simulink library "myLibrary"  (R2023b)
settings: Solver=VariableStepAuto  StartTime=0.0  StopTime=10.0  RelTol=1e-3
undefined symbols (not defined in the file): Cac_n1, ctrl1, Da, Discrete, dtha, ee_sli_rtmsupport, FA, gcbh, Ha, Ini, init_DCline, init_IPC, init_line, init_load, init_SG, init_shunt, init_TH, init_trafo, init_VSC, initMachineBlocks, Ka, Lf, Llkd_pu, Llkq1_pu, magnitude, NET, P, plots_step, q0, Rac_n1, Radd, Rkd_pu, Rkq1_pu, Rload_add, sim_config, sps_rtmsupport, spsSteamTurbineModel, T_DC_NET, T_global, T_IPC, T_load, T_NET, T_SG, T_shunt, T_STATCOM, T_TH, T_trafo, T_VSC, Ts, tstep, Udiff_a, V1
libraries: spsSeriesRLCBranchLib x105, eeGeneralControl x72, $bdroot x70, spsCurrentMeasurementLib x48, spsParallelRLCBranchLib x39, spsVoltageMeasurementLib x33, spsControlledVoltageSourceLib x27, spsFirstOrderFilterLib x16, dspsigops x6, spsThreePhaseVIMeasurementLib x5, spsPLL3phLib x4, spsThreePhaseBreakerLib x3
(part 2 of 12)

== system myLibrary/HVDC_line ==
  Current Measurement : spsCurrentMeasurementLib/Current Measurement  PhasorSimulation=off  OutputType=Complex  PSBequivalent=0
  Current Measurement1 : Subsystem  DialogController=POWERSYS.PowerSysDialog  LoadFcn=sps_rtmsupport('LoadFcn',gcbh);  StartFcn=sps_rtmsupport('StartFcn',gcbh);  StopFcn=sps_rtmsupport('StopFcn',gcbh);  mask(Current Measurement){PhasorSimulation=off, OutputType=Complex, PSBequivalent=0}
      mask prompts: PhasorSimulation "Phasor simulation"; OutputType "Output signal :"; PSBequivalent "Equivalent circuit"
      mask help: Ideal current measurement. The Output signal parameter is disabled when the block is not used in a phasor simulation. The phasor simulation is activated by a Powergui block placed in the model.
      mask init:
      | block = gcb;
      | powericon('psbloadfunction',block,'Measurement Block','Initialize');
      | WantBlockChoice = powericon('MeasurementBlockInit',block);
      | powericon('SetInternalModels','set',block,WantBlockChoice);
      | power_initmask();
      settings: LibrarySourceBlock=sps_lib/Sensors and Measurements/Current Measurement  CopyFcn=sps_rtmsupport('CopyFcn',gcbh); powericon('psbloadfunction',gcb,'Measurement Block','UpdateGotoTag');  DeleteFcn=sps_rtmsupport('DeleteFcn',gcbh);  UndoDeleteFcn=sps_rtmsupport('UndoDeleteFcn',gcbh);  ModelCloseFcn=sps_rtmsupport('ModelCloseFcn',gcbh);  PreSaveFcn=sps_rtmsupport('PreSaveFcn',gcbh);  PostSaveFcn=sps_rtmsupport('PostSaveFcn',gcbh);  PreCopyFcn=sps_rtmsupport('PreCopyFcn',gcbh);  OpenFcn=sps_rtmsupport('OpenFcn',gcbh, [1 -2]);  CloseFcn=sps_rtmsupport('CloseFcn',gcbh);  PreDeleteFcn=sps_rtmsupport('PreDeleteFcn',gcbh);
      settings: NameChangeFcn=|
      | sps_rtmsupport('NameChangeFcn',gcbh);
      | powericon('SetNewGotoTag',[gcb,'/source'],-2);
      mask Help: helpview(psbhelp);
      mask TypeOptions OutputType: Complex | Real-Imag | Magnitude-Angle | Magnitude
  Current Measurement2 : Subsystem  DialogController=POWERSYS.PowerSysDialog  LoadFcn=sps_rtmsupport('LoadFcn',gcbh);  StartFcn=sps_rtmsupport('StartFcn',gcbh);  StopFcn=sps_rtmsupport('StopFcn',gcbh);  mask(Current Measurement){PhasorSimulation=off, OutputType=Complex, PSBequivalent=0}
      mask prompts: PhasorSimulation "Phasor simulation"; OutputType "Output signal :"; PSBequivalent "Equivalent circuit"
      mask help: Ideal current measurement. The Output signal parameter is disabled when the block is not used in a phasor simulation. The phasor simulation is activated by a Powergui block placed in the model.
      mask init: same as myLibrary/HVDC_line/Current Measurement1
      settings: LibrarySourceBlock=sps_lib/Sensors and Measurements/Current Measurement  CopyFcn=sps_rtmsupport('CopyFcn',gcbh); powericon('psbloadfunction',gcb,'Measurement Block','UpdateGotoTag');  DeleteFcn=sps_rtmsupport('DeleteFcn',gcbh);  UndoDeleteFcn=sps_rtmsupport('UndoDeleteFcn',gcbh);  ModelCloseFcn=sps_rtmsupport('ModelCloseFcn',gcbh);  PreSaveFcn=sps_rtmsupport('PreSaveFcn',gcbh);  PostSaveFcn=sps_rtmsupport('PostSaveFcn',gcbh);  PreCopyFcn=sps_rtmsupport('PreCopyFcn',gcbh);  OpenFcn=sps_rtmsupport('OpenFcn',gcbh, [1 -2]);  CloseFcn=sps_rtmsupport('CloseFcn',gcbh);  PreDeleteFcn=sps_rtmsupport('PreDeleteFcn',gcbh);
      settings: NameChangeFcn=|
      | sps_rtmsupport('NameChangeFcn',gcbh);
      | powericon('SetNewGotoTag',[gcb,'/source'],-2);
      mask Help: helpview(psbhelp);
      mask TypeOptions OutputType: Complex | Real-Imag | Magnitude-Angle | Magnitude
  Scope : Scope  NumInputPorts=3
  Series RLC Branch1 : PMComponent  DialogController=POWERSYS.PowerSysDialog  LoadFcn=sps_rtmsupport('LoadFcn',gcbh);  StartFcn=sps_rtmsupport('StartFcn',gcbh);  StopFcn=sps_rtmsupport('StopFcn',gcbh);  PhysicalDomain=powersysdomain  LeftPortType=p1  RightPortType=p1  LConnTagsString=__new0  RConnTagsString=__new0  mask(Series RLC Branch){BranchType=C, Resistance=1, Inductance=1e-3, SetiL0=off, InitialCurrent=0, Capacitance=T.C, Setx0=on, InitialVoltage=ini.V1, Measurements=None}
      mask prompts: BranchType "Branch type:"; Resistance "Resistance (Ohms):"; Inductance "Inductance (H):"; SetiL0 "Set the initial inductor current"; InitialCurrent "Inductor initial current (A):"; Capacitance "Capacitance (F):"; Setx0 "Set the initial capacitor voltage"; InitialVoltage "Capacitor initial voltage (V):"
      mask help:
      | Implements a series branch of RLC elements.
      | Use the 'Branch type' parameter to add or remove elements from the branch.
      mask init:
      | [s1,s2,s3,s4,r1,r2,l1,l2,c1,c2,c3,c4] = powericon('Series RLC Branch',Resistance,Inductance,Capacitance,BranchType);
      | powericon('RLCCback',gcb)
      | power_initmask();
      settings: LibrarySourceBlock=spsSeriesRLCBranchLib/Series RLC Branch  CopyFcn=sps_rtmsupport('CopyFcn',gcbh);  DeleteFcn=sps_rtmsupport('DeleteFcn',gcbh);  UndoDeleteFcn=sps_rtmsupport('UndoDeleteFcn',gcbh);  ModelCloseFcn=sps_rtmsupport('ModelCloseFcn',gcbh);  PreSaveFcn=sps_rtmsupport('PreSaveFcn',gcbh);  PostSaveFcn=sps_rtmsupport('PostSaveFcn',gcbh);  NameChangeFcn=sps_rtmsupport('NameChangeFcn',gcbh);  PreCopyFcn=sps_rtmsupport('PreCopyFcn',gcbh);  OpenFcn=sps_rtmsupport('OpenFcn',gcbh, [1 4 7 9]);  CloseFcn=sps_rtmsupport('CloseFcn',gcbh);  PreDeleteFcn=sps_rtmsupport('PreDeleteFcn',gcbh);
      mask Help: helpview(psbhelp);
      mask TypeOptions BranchType: RLC | R | L | C | RL | RC | LC | Open circuit
      mask Callback BranchType: powericon('RLCCback',gcb)
      mask Callback Resistance: powericon('RLCCback',gcb)
      mask Callback Inductance: powericon('RLCCback',gcb)
      mask Callback SetiL0: powericon('RLCCback',gcb)
      mask Callback Capacitance: powericon('RLCCback',gcb)
      mask Callback Setx0: powericon('RLCCback',gcb)
      mask TypeOptions Measurements: None | Branch voltage | Branch current | Branch voltage and current
      mask Display:
      | plot(s1,s2,s3,s4,r1,r2*1.5,l1,l2*1.5,c1,c2*1.5,c3,c4*1.5)
      | color('red')
      | port_label('LConn',1,'+')
  Series RLC Branch4 : spsSeriesRLCBranchLib/Series RLC Branch  LConnTagsString=__new0  RConnTagsString=__new0  BranchType=C  Resistance=1  Inductance=1e-3  SetiL0=off  InitialCurrent=0  Capacitance=T.C  Setx0=on  InitialVoltage=ini.V2  Measurements=None
  Series RLC Branch6 : spsSeriesRLCBranchLib/Series RLC Branch  LConnTagsString=__new0  RConnTagsString=__new0  BranchType=RL  Resistance=T.Ra  Inductance=T.La  SetiL0=on  InitialCurrent=ini.Ia  Capacitance=P.C  Setx0=on  InitialVoltage=P.C  Measurements=None
  Series RLC Branch7 : spsSeriesRLCBranchLib/Series RLC Branch  LConnTagsString=__new0  RConnTagsString=__new0  BranchType=RL  Resistance=T.Rc  Inductance=T.Lc  SetiL0=on  InitialCurrent=ini.Ic  Capacitance=P.C  Setx0=on  InitialVoltage=P.C  Measurements=None
  Series RLC Branch8 : spsSeriesRLCBranchLib/Series RLC Branch  LConnTagsString=__new0  RConnTagsString=__new0  BranchType=RL  Resistance=T.Rb  Inductance=T.Lb  SetiL0=on  InitialCurrent=ini.Ib  Capacitance=P.C  Setx0=on  InitialVoltage=P.C  Measurements=None
  Vdc+2 : PMIOPort  Side=Right
  Vcd+1 : PMIOPort  Port=2  Side=Left
  Vdc-1 : PMIOPort  Port=3  Side=Left
  Vdc-2 : PMIOPort  Port=4  Side=Right
  wires:
  Current Measurement/1 -> Scope/1
  Current Measurement1/1(i) -> Scope/2
  Current Measurement2/1(i) -> Scope/3
  connections:
  Series RLC Branch4/LConn1 -- Current Measurement1/RConn1 -- Current Measurement/RConn1 -- Current Measurement2/RConn1 -- Vdc+2/RConn1
  Series RLC Branch1/LConn1 -- Vcd+1/RConn1 -- Series RLC Branch7/LConn1 -- Series RLC Branch6/LConn1 -- Series RLC Branch8/LConn1
  Vdc-1/RConn1 -- Vdc-2/RConn1 -- Series RLC Branch4/RConn1 -- Series RLC Branch1/RConn1
  Current Measurement/LConn1 -- Series RLC Branch6/RConn1
  Series RLC Branch8/RConn1 -- Current Measurement1/LConn1
  Current Measurement2/LConn1 -- Series RLC Branch7/RConn1

== system myLibrary/Load ==
  Parallel RLC Branch : spsParallelRLCBranchLib/Parallel RLC Branch  LConnTagsString=a  RConnTagsString=__new0  BranchType=R  Resistance=T.R  Inductance=P.L  SetiL0=on  InitialCurrent=Ini.Ia*10  Capacitance=1e-6  Setx0=off  InitialVoltage=0  Measurements=None
  Parallel RLC Branch1 : spsParallelRLCBranchLib/Parallel RLC Branch  LConnTagsString=a  RConnTagsString=__new0  BranchType=R  Resistance=T.R  Inductance=P.L  SetiL0=on  InitialCurrent=Ini.Ia*10  Capacitance=1e-6  Setx0=off  InitialVoltage=0  Measurements=None
  Parallel RLC Branch2 : spsParallelRLCBranchLib/Parallel RLC Branch  LConnTagsString=a  RConnTagsString=__new0  BranchType=L  Resistance=P.R  Inductance=T.L  SetiL0=on  InitialCurrent=ini.Ib  Capacitance=1e-6  Setx0=off  InitialVoltage=0  Measurements=None
  Parallel RLC Branch3 : spsParallelRLCBranchLib/Parallel RLC Branch  LConnTagsString=a  RConnTagsString=__new0  BranchType=L  Resistance=P.R  Inductance=T.L  SetiL0=on  InitialCurrent=ini.Ia  Capacitance=1e-6  Setx0=off  InitialVoltage=0  Measurements=None
  Parallel RLC Branch4 : spsParallelRLCBranchLib/Parallel RLC Branch  LConnTagsString=a  RConnTagsString=__new0  BranchType=R  Resistance=T.R  Inductance=P.L  SetiL0=on  InitialCurrent=Ini.Ia*10  Capacitance=1e-6  Setx0=off  InitialVoltage=0  Measurements=None
  Parallel RLC Branch5 : spsParallelRLCBranchLib/Parallel RLC Branch  LConnTagsString=a  RConnTagsString=__new0  BranchType=L  Resistance=P.R  Inductance=T.L  SetiL0=on  InitialCurrent=ini.Ic  Capacitance=1e-6  Setx0=off  InitialVoltage=0  Measurements=None
  A : PMIOPort  Side=Left
  B : PMIOPort  Port=2  Side=Left
  C : PMIOPort  Port=3  Side=Left
  connections:
  Parallel RLC Branch2/LConn1 -- Parallel RLC Branch1/RConn1 -- Parallel RLC Branch3/LConn1 -- Parallel RLC Branch/RConn1 -- Parallel RLC Branch4/RConn1 -- Parallel RLC Branch5/LConn1
  A/RConn1 -- Parallel RLC Branch3/RConn1 -- Parallel RLC Branch/LConn1
  Parallel RLC Branch1/LConn1 -- B/RConn1 -- Parallel RLC Branch2/RConn1
  C/RConn1 -- Parallel RLC Branch5/RConn1 -- Parallel RLC Branch4/LConn1

== system myLibrary/LoadC ==
  Parallel RLC Branch : spsParallelRLCBranchLib/Parallel RLC Branch  LConnTagsString=a  RConnTagsString=__new0  BranchType=R  Resistance=T.R  Inductance=P.L  SetiL0=on  InitialCurrent=Ini.Ia*10  Capacitance=1e-6  Setx0=off  InitialVoltage=0  Measurements=None
  Parallel RLC Branch1 : spsParallelRLCBranchLib/Parallel RLC Branch  LConnTagsString=a  RConnTagsString=__new0  BranchType=R  Resistance=T.R  Inductance=P.L  SetiL0=on  InitialCurrent=Ini.Ia*10  Capacitance=1e-6  Setx0=off  InitialVoltage=0  Measurements=None
  Parallel RLC Branch2 : spsParallelRLCBranchLib/Parallel RLC Branch  LConnTagsString=a  RConnTagsString=__new0  BranchType=C  Resistance=T.R  Inductance=P.L  SetiL0=on  InitialCurrent=Ini.Ia*10  Capacitance=T.C  Setx0=on  InitialVoltage=ini.Va  Measurements=None
  Parallel RLC Branch3 : spsParallelRLCBranchLib/Parallel RLC Branch  LConnTagsString=a  RConnTagsString=__new0  BranchType=C  Resistance=T.R  Inductance=P.L  SetiL0=on  InitialCurrent=Ini.Ia*10  Capacitance=T.C  Setx0=on  InitialVoltage=ini.Vb  Measurements=None
  Parallel RLC Branch4 : spsParallelRLCBranchLib/Parallel RLC Branch  LConnTagsString=a  RConnTagsString=__new0  BranchType=R  Resistance=T.R  Inductance=P.L  SetiL0=on  InitialCurrent=Ini.Ia*10  Capacitance=1e-6  Setx0=off  InitialVoltage=0  Measurements=None
  Parallel RLC Branch5 : spsParallelRLCBranchLib/Parallel RLC Branch  LConnTagsString=a  RConnTagsString=__new0  BranchType=C  Resistance=T.R  Inductance=P.L  SetiL0=on  InitialCurrent=Ini.Ia*10  Capacitance=T.C  Setx0=on  InitialVoltage=ini.Vc  Measurements=None
  A : PMIOPort  Side=Left
  B : PMIOPort  Port=2  Side=Left
  C : PMIOPort  Port=3  Side=Left
  connections:
  Parallel RLC Branch1/RConn1 -- Parallel RLC Branch3/RConn1 -- Parallel RLC Branch2/RConn1 -- Parallel RLC Branch/RConn1 -- Parallel RLC Branch5/RConn1 -- Parallel RLC Branch4/RConn1
  A/RConn1 -- Parallel RLC Branch2/LConn1 -- Parallel RLC Branch/LConn1
  Parallel RLC Branch1/LConn1 -- Parallel RLC Branch3/LConn1 -- B/RConn1
  C/RConn1 -- Parallel RLC Branch5/LConn1 -- Parallel RLC Branch4/LConn1

== system myLibrary/LoadC_Rstep ==
  Parallel RLC Branch : spsParallelRLCBranchLib/Parallel RLC Branch  LConnTagsString=a  RConnTagsString=__new0  BranchType=R  Resistance=T.R  Inductance=P.L  SetiL0=on  InitialCurrent=Ini.Ia*10  Capacitance=1e-6  Setx0=off  InitialVoltage=0  Measurements=None
  Parallel RLC Branch1 : spsParallelRLCBranchLib/Parallel RLC Branch  LConnTagsString=a  RConnTagsString=__new0  BranchType=R  Resistance=T.R  Inductance=P.L  SetiL0=on  InitialCurrent=Ini.Ia*10  Capacitance=1e-6  Setx0=off  InitialVoltage=0  Measurements=None
  Parallel RLC Branch10 : spsParallelRLCBranchLib/Parallel RLC Branch  LConnTagsString=a  RConnTagsString=__new0  BranchType=R  Resistance=Rload_add  Inductance=P.L  SetiL0=on  InitialCurrent=Ini.Ia*10  Capacitance=1e-6  Setx0=off  InitialVoltage=0  Measurements=None
  Parallel RLC Branch2 : spsParallelRLCBranchLib/Parallel RLC Branch  LConnTagsString=a  RConnTagsString=__new0  BranchType=C  Resistance=T.R  Inductance=P.L  SetiL0=on  InitialCurrent=Ini.Ia*10  Capacitance=T.C  Setx0=on  InitialVoltage=ini.Va  Measurements=None
  Parallel RLC Branch3 : spsParallelRLCBranchLib/Parallel RLC Branch  LConnTagsString=a  RConnTagsString=__new0  BranchType=C  Resistance=T.R  Inductance=P.L  SetiL0=on  InitialCurrent=Ini.Ia*10  Capacitance=T.C  Setx0=on  InitialVoltage=ini.Vb  Measurements=None
  Parallel RLC Branch4 : spsParallelRLCBranchLib/Parallel RLC Branch  LConnTagsString=a  RConnTagsString=__new0  BranchType=R  Resistance=T.R  Inductance=P.L  SetiL0=on  InitialCurrent=Ini.Ia*10  Capacitance=1e-6  Setx0=off  InitialVoltage=0  Measurements=None
  Parallel RLC Branch5 : spsParallelRLCBranchLib/Parallel RLC Branch  LConnTagsString=a  RConnTagsString=__new0  BranchType=C  Resistance=T.R  Inductance=P.L  SetiL0=on  InitialCurrent=Ini.Ia*10  Capacitance=T.C  Setx0=on  InitialVoltage=ini.Vc  Measurements=None
  Parallel RLC Branch6 : spsParallelRLCBranchLib/Parallel RLC Branch  LConnTagsString=a  RConnTagsString=__new0  BranchType=R  Resistance=Rload_add  Inductance=P.L  SetiL0=on  InitialCurrent=Ini.Ia*10  Capacitance=1e-6  Setx0=off  InitialVoltage=0  Measurements=None
  Parallel RLC Branch7 : spsParallelRLCBranchLib/Parallel RLC Branch  LConnTagsString=a  RConnTagsString=__new0  BranchType=R  Resistance=Rload_add  Inductance=P.L  SetiL0=on  InitialCurrent=Ini.Ia*10  Capacitance=1e-6  Setx0=off  InitialVoltage=0  Measurements=None
  Three-Phase Breaker : spsThreePhaseBreakerLib/Three-Phase Breaker  InitialState=open  SwitchA=on  SwitchB=on  SwitchC=on  SwitchTimes=[tstep 1e6]  External=off  BreakerResistance=1e-10  SnubberResistance=inf  SnubberCapacitance=inf  Measurements=None
  A : PMIOPort  Side=Left
  B : PMIOPort  Port=2  Side=Left
  C : PMIOPort  Port=3  Side=Left
  connections:
  Three-Phase Breaker/RConn3 -- Parallel RLC Branch10/LConn1
  Three-Phase Breaker/RConn2 -- Parallel RLC Branch7/LConn1
  Three-Phase Breaker/RConn1 -- Parallel RLC Branch6/LConn1
  Parallel RLC Branch10/RConn1 -- Parallel RLC Branch7/RConn1 -- Parallel RLC Branch6/RConn1 -- Parallel RLC Branch4/RConn1 -- Parallel RLC Branch2/RConn1 -- Parallel RLC Branch/RConn1 -- Parallel RLC Branch3/RConn1 -- Parallel RLC Branch1/RConn1 -- Parallel RLC Branch5/RConn1
  Parallel RLC Branch4/LConn1 -- Parallel RLC Branch5/LConn1 -- C/RConn1 -- Three-Phase Breaker/LConn3
  Parallel RLC Branch1/LConn1 -- Parallel RLC Branch3/LConn1 -- B/RConn1 -- Three-Phase Breaker/LConn2
  Parallel RLC Branch/LConn1 -- Parallel RLC Branch2/LConn1 -- A/RConn1 -- Three-Phase Breaker/LConn1

== system myLibrary/Load_R ==
  Parallel RLC Branch : spsParallelRLCBranchLib/Parallel RLC Branch  LConnTagsString=a  RConnTagsString=__new0  BranchType=R  Resistance=T.R  Inductance=P.L  SetiL0=on  InitialCurrent=Ini.Ia*10  Capacitance=1e-6  Setx0=off  InitialVoltage=0  Measurements=None
  Parallel RLC Branch1 : spsParallelRLCBranchLib/Parallel RLC Branch  LConnTagsString=a  RConnTagsString=__new0  BranchType=R  Resistance=T.R  Inductance=P.L  SetiL0=on  InitialCurrent=Ini.Ia*10  Capacitance=1e-6  Setx0=off  InitialVoltage=0  Measurements=None
  Parallel RLC Branch4 : spsParallelRLCBranchLib/Parallel RLC Branch  LConnTagsString=a  RConnTagsString=__new0  BranchType=R  Resistance=T.R  Inductance=P.L  SetiL0=on  InitialCurrent=Ini.Ia*10  Capacitance=1e-6  Setx0=off  InitialVoltage=0  Measurements=None
  A : PMIOPort  Side=Left
  B : PMIOPort  Port=2  Side=Left
  C : PMIOPort  Port=3  Side=Left
  connections:
  Parallel RLC Branch1/RConn1 -- Parallel RLC Branch4/RConn1 -- Parallel RLC Branch/RConn1
  Parallel RLC Branch/LConn1 -- A/RConn1
  Parallel RLC Branch1/LConn1 -- B/RConn1
  Parallel RLC Branch4/LConn1 -- C/RConn1

== system myLibrary/Load_R_Rstep ==
  Parallel RLC Branch : spsParallelRLCBranchLib/Parallel RLC Branch  LConnTagsString=a  RConnTagsString=__new0  BranchType=R  Resistance=T.R  Inductance=P.L  SetiL0=on  InitialCurrent=Ini.Ia*10  Capacitance=1e-6  Setx0=off  InitialVoltage=0  Measurements=None
  Parallel RLC Branch1 : spsParallelRLCBranchLib/Parallel RLC Branch  LConnTagsString=a  RConnTagsString=__new0  BranchType=R  Resistance=T.R  Inductance=P.L  SetiL0=on  InitialCurrent=Ini.Ia*10  Capacitance=1e-6  Setx0=off  InitialVoltage=0  Measurements=None
  Parallel RLC Branch10 : spsParallelRLCBranchLib/Parallel RLC Branch  LConnTagsString=a  RConnTagsString=__new0  BranchType=R  Resistance=Rload_add  Inductance=P.L  SetiL0=on  InitialCurrent=Ini.Ia*10  Capacitance=1e-6  Setx0=off  InitialVoltage=0  Measurements=None
  Parallel RLC Branch4 : spsParallelRLCBranchLib/Parallel RLC Branch  LConnTagsString=a  RConnTagsString=__new0  BranchType=R  Resistance=T.R  Inductance=P.L  SetiL0=on  InitialCurrent=Ini.Ia*10  Capacitance=1e-6  Setx0=off  InitialVoltage=0  Measurements=None
  Parallel RLC Branch6 : spsParallelRLCBranchLib/Parallel RLC Branch  LConnTagsString=a  RConnTagsString=__new0  BranchType=R  Resistance=Rload_add  Inductance=P.L  SetiL0=on  InitialCurrent=Ini.Ia*10  Capacitance=1e-6  Setx0=off  InitialVoltage=0  Measurements=None
  Parallel RLC Branch7 : spsParallelRLCBranchLib/Parallel RLC Branch  LConnTagsString=a  RConnTagsString=__new0  BranchType=R  Resistance=Rload_add  Inductance=P.L  SetiL0=on  InitialCurrent=Ini.Ia*10  Capacitance=1e-6  Setx0=off  InitialVoltage=0  Measurements=None
  Three-Phase Breaker : spsThreePhaseBreakerLib/Three-Phase Breaker  InitialState=open  SwitchA=on  SwitchB=on  SwitchC=on  SwitchTimes=[tstep 1e6]  External=off  BreakerResistance=1e-10  SnubberResistance=inf  SnubberCapacitance=inf  Measurements=None
  A : PMIOPort  Side=Left
  B : PMIOPort  Port=2  Side=Left
  C : PMIOPort  Port=3  Side=Left
  connections:
  Three-Phase Breaker/LConn1 -- Parallel RLC Branch/LConn1 -- A/RConn1
  Parallel RLC Branch1/LConn1 -- Three-Phase Breaker/LConn2 -- B/RConn1
  Three-Phase Breaker/LConn3 -- Parallel RLC Branch4/LConn1 -- C/RConn1
  Parallel RLC Branch1/RConn1 -- Parallel RLC Branch/RConn1 -- Parallel RLC Branch6/RConn1 -- Parallel RLC Branch7/RConn1 -- Parallel RLC Branch10/RConn1 -- Parallel RLC Branch4/RConn1
  Three-Phase Breaker/RConn1 -- Parallel RLC Branch6/LConn1
  Three-Phase Breaker/RConn2 -- Parallel RLC Branch7/LConn1
  Three-Phase Breaker/RConn3 -- Parallel RLC Branch10/LConn1

== system myLibrary/Load_Rstep ==
  Parallel RLC Branch : spsParallelRLCBranchLib/Parallel RLC Branch  LConnTagsString=a  RConnTagsString=__new0  BranchType=R  Resistance=T.R  Inductance=P.L  SetiL0=on  InitialCurrent=Ini.Ia*10  Capacitance=1e-6  Setx0=off  InitialVoltage=0  Measurements=None
  Parallel RLC Branch1 : spsParallelRLCBranchLib/Parallel RLC Branch  LConnTagsString=a  RConnTagsString=__new0  BranchType=R  Resistance=T.R  Inductance=P.L  SetiL0=on  InitialCurrent=Ini.Ia*10  Capacitance=1e-6  Setx0=off  InitialVoltage=0  Measurements=None
  Parallel RLC Branch10 : spsParallelRLCBranchLib/Parallel RLC Branch  LConnTagsString=a  RConnTagsString=__new0  BranchType=R  Resistance=Rload_add  Inductance=P.L  SetiL0=on  InitialCurrent=Ini.Ia*10  Capacitance=1e-6  Setx0=off  InitialVoltage=0  Measurements=None
  Parallel RLC Branch2 : spsParallelRLCBranchLib/Parallel RLC Branch  LConnTagsString=a  RConnTagsString=__new0  BranchType=L  Resistance=P.R  Inductance=T.L  SetiL0=on  InitialCurrent=ini.Ib  Capacitance=1e-6  Setx0=off  InitialVoltage=0  Measurements=None
  Parallel RLC Branch3 : spsParallelRLCBranchLib/Parallel RLC Branch  LConnTagsString=a  RConnTagsString=__new0  BranchType=L  Resistance=P.R  Inductance=T.L  SetiL0=on  InitialCurrent=ini.Ia  Capacitance=1e-6  Setx0=off  InitialVoltage=0  Measurements=None
  Parallel RLC Branch4 : spsParallelRLCBranchLib/Parallel RLC Branch  LConnTagsString=a  RConnTagsString=__new0  BranchType=R  Resistance=T.R  Inductance=P.L  SetiL0=on  InitialCurrent=Ini.Ia*10  Capacitance=1e-6  Setx0=off  InitialVoltage=0  Measurements=None
  Parallel RLC Branch5 : spsParallelRLCBranchLib/Parallel RLC Branch  LConnTagsString=a  RConnTagsString=__new0  BranchType=L  Resistance=P.R  Inductance=T.L  SetiL0=on  InitialCurrent=ini.Ic  Capacitance=1e-6  Setx0=off  InitialVoltage=0  Measurements=None
  Parallel RLC Branch6 : spsParallelRLCBranchLib/Parallel RLC Branch  LConnTagsString=a  RConnTagsString=__new0  BranchType=R  Resistance=Rload_add  Inductance=P.L  SetiL0=on  InitialCurrent=Ini.Ia*10  Capacitance=1e-6  Setx0=off  InitialVoltage=0  Measurements=None
  Parallel RLC Branch7 : spsParallelRLCBranchLib/Parallel RLC Branch  LConnTagsString=a  RConnTagsString=__new0  BranchType=R  Resistance=Rload_add  Inductance=P.L  SetiL0=on  InitialCurrent=Ini.Ia*10  Capacitance=1e-6  Setx0=off  InitialVoltage=0  Measurements=None
  Three-Phase Breaker : spsThreePhaseBreakerLib/Three-Phase Breaker  InitialState=open  SwitchA=on  SwitchB=on  SwitchC=on  SwitchTimes=[tstep 1e6]  External=off  BreakerResistance=1e-10  SnubberResistance=inf  SnubberCapacitance=inf  Measurements=None
  A : PMIOPort  Side=Left
  B : PMIOPort  Port=2  Side=Left
  C : PMIOPort  Port=3  Side=Left
  connections:
  Three-Phase Breaker/LConn1 -- A/RConn1 -- Parallel RLC Branch3/RConn1 -- Parallel RLC Branch/LConn1
  Parallel RLC Branch1/LConn1 -- Three-Phase Breaker/LConn2 -- B/RConn1 -- Parallel RLC Branch2/RConn1
  Three-Phase Breaker/LConn3 -- C/RConn1 -- Parallel RLC Branch5/RConn1 -- Parallel RLC Branch4/LConn1
  Parallel RLC Branch2/LConn1 -- Parallel RLC Branch1/RConn1 -- Parallel RLC Branch3/LConn1 -- Parallel RLC Branch/RConn1 -- Parallel RLC Branch4/RConn1 -- Parallel RLC Branch5/LConn1 -- Parallel RLC Branch6/RConn1 -- Parallel RLC Branch7/RConn1 -- Parallel RLC Branch10/RConn1
  Three-Phase Breaker/RConn1 -- Parallel RLC Branch6/LConn1
  Three-Phase Breaker/RConn2 -- Parallel RLC Branch7/LConn1
  Three-Phase Breaker/RConn3 -- Parallel RLC Branch10/LConn1

== system myLibrary/PI_line ==
  Series RLC Branch : spsSeriesRLCBranchLib/Series RLC Branch  LConnTagsString=__new0  RConnTagsString=__new0  BranchType=C  Resistance=1  Inductance=1e-3  SetiL0=off  InitialCurrent=0  Capacitance=T.C  Setx0=on  InitialVoltage=ini.Va1  Measurements=None
  Series RLC Branch1 : spsSeriesRLCBranchLib/Series RLC Branch  LConnTagsString=__new0  RConnTagsString=__new0  BranchType=C  Resistance=1  Inductance=1e-3  SetiL0=off  InitialCurrent=0  Capacitance=T.C  Setx0=on  InitialVoltage=ini.Vb1  Measurements=None
  Series RLC Branch2 : spsSeriesRLCBranchLib/Series RLC Branch  LConnTagsString=__new0  RConnTagsString=__new0  BranchType=C  Resistance=1  Inductance=1e-3  SetiL0=off  InitialCurrent=0  Capacitance=T.C  Setx0=on  InitialVoltage=ini.Vc1  Measurements=None
  Series RLC Branch3 : spsSeriesRLCBranchLib/Series RLC Branch  LConnTagsString=__new0  RConnTagsString=__new0  BranchType=C  Resistance=1  Inductance=1e-3  SetiL0=off  InitialCurrent=0  Capacitance=T.C  Setx0=on  InitialVoltage=ini.Va2  Measurements=None
  Series RLC Branch4 : spsSeriesRLCBranchLib/Series RLC Branch  LConnTagsString=__new0  RConnTagsString=__new0  BranchType=C  Resistance=1  Inductance=1e-3  SetiL0=off  InitialCurrent=0  Capacitance=T.C  Setx0=on  InitialVoltage=ini.Vb2  Measurements=None
  Series RLC Branch5 : spsSeriesRLCBranchLib/Series RLC Branch  LConnTagsString=__new0  RConnTagsString=__new0  BranchType=C  Resistance=1  Inductance=1e-3  SetiL0=off  InitialCurrent=0  Capacitance=T.C  Setx0=on  InitialVoltage=ini.Vc2  Measurements=None
  Series RLC Branch6 : spsSeriesRLCBranchLib/Series RLC Branch  LConnTagsString=__new0  RConnTagsString=__new0  BranchType=RL  Resistance=T.R  Inductance=T.L  SetiL0=off  InitialCurrent=ini.Ia  Capacitance=P.C  Setx0=on  InitialVoltage=P.C  Measurements=None
  Series RLC Branch7 : spsSeriesRLCBranchLib/Series RLC Branch  LConnTagsString=__new0  RConnTagsString=__new0  BranchType=RL  Resistance=T.R  Inductance=T.L  SetiL0=on  InitialCurrent=ini.Ic  Capacitance=P.C  Setx0=on  InitialVoltage=P.C  Measurements=None
  Series RLC Branch8 : spsSeriesRLCBranchLib/Series RLC Branch  LConnTagsString=__new0  RConnTagsString=__new0  BranchType=RL  Resistance=T.R  Inductance=T.L  SetiL0=on  InitialCurrent=ini.Ib  Capacitance=P.C  Setx0=on  InitialVoltage=P.C  Measurements=None
  A1 : PMIOPort  Side=Left
  B1 : PMIOPort  Port=2  Side=Left
  C1 : PMIOPort  Port=3  Side=Left
  A2 : PMIOPort  Port=4  Side=Right
  B2 : PMIOPort  Port=5  Side=Right
  C2 : PMIOPort  Port=6  Side=Right
  connections:
  C2/RConn1 -- Series RLC Branch7/RConn1 -- Series RLC Branch5/LConn1
  B2/RConn1 -- Series RLC Branch8/RConn1 -- Series RLC Branch4/LConn1
  Series RLC Branch3/LConn1 -- Series RLC Branch6/RConn1 -- A2/RConn1
  C1/RConn1 -- Series RLC Branch7/LConn1 -- Series RLC Branch2/LConn1
  Series RLC Branch6/LConn1 -- A1/RConn1 -- Series RLC Branch/LConn1
  Series RLC Branch8/LConn1 -- B1/RConn1 -- Series RLC Branch1/LConn1
  Series RLC Branch2/RConn1 -- Series RLC Branch/RConn1 -- Series RLC Branch1/RConn1
  Series RLC Branch5/RConn1 -- Series RLC Branch4/RConn1 -- Series RLC Branch3/RConn1

== system myLibrary/RC ==
  RLC1 : spsSeriesRLCBranchLib/Series RLC Branch  LConnTagsString=__new0  RConnTagsString=__new0  BranchType=RC  Resistance=T.R/T.Zbpu_l2g  Inductance=T.L/T.Zbpu_l2g  SetiL0=on  InitialCurrent=ini.iL_a  Capacitance=T.C*T.Zbpu_l2g  Setx0=on  InitialVoltage=ini.vC_a  Measurements=None
  RLC2 : spsSeriesRLCBranchLib/Series RLC Branch  LConnTagsString=__new0  RConnTagsString=__new0  BranchType=RC  Resistance=T.R/T.Zbpu_l2g  Inductance=T.L/T.Zbpu_l2g  SetiL0=on  InitialCurrent=ini.iL_b  Capacitance=T.C*T.Zbpu_l2g  Setx0=on  InitialVoltage=ini.vC_b  Measurements=None
  RLC3 : spsSeriesRLCBranchLib/Series RLC Branch  LConnTagsString=__new0  RConnTagsString=__new0  BranchType=RC  Resistance=T.R/T.Zbpu_l2g  Inductance=T.L/T.Zbpu_l2g  SetiL0=on  InitialCurrent=ini.iL_c  Capacitance=T.C*T.Zbpu_l2g  Setx0=on  InitialVoltage=ini.vC_c  Measurements=None
  A : PMIOPort  Side=Left
  B : PMIOPort  Port=2  Side=Left
  C : PMIOPort  Port=3  Side=Left
  connections:
  RLC2/RConn1 -- RLC3/RConn1 -- RLC1/RConn1
  RLC3/LConn1 -- C/RConn1
  RLC2/LConn1 -- B/RConn1
  RLC1/LConn1 -- A/RConn1

== system myLibrary/RLC ==
  RLC1 : spsSeriesRLCBranchLib/Series RLC Branch  LConnTagsString=__new0  RConnTagsString=__new0  BranchType=RLC  Resistance=T.R/T.Zbpu_l2g  Inductance=T.L/T.Zbpu_l2g  SetiL0=on  InitialCurrent=ini.iL_a  Capacitance=T.C*T.Zbpu_l2g  Setx0=on  InitialVoltage=ini.vC_a  Measurements=None
  RLC2 : spsSeriesRLCBranchLib/Series RLC Branch  LConnTagsString=__new0  RConnTagsString=__new0  BranchType=RLC  Resistance=T.R/T.Zbpu_l2g  Inductance=T.L/T.Zbpu_l2g  SetiL0=on  InitialCurrent=ini.iL_b  Capacitance=T.C*T.Zbpu_l2g  Setx0=on  InitialVoltage=ini.vC_b  Measurements=None
  RLC3 : spsSeriesRLCBranchLib/Series RLC Branch  LConnTagsString=__new0  RConnTagsString=__new0  BranchType=RLC  Resistance=T.R/T.Zbpu_l2g  Inductance=T.L/T.Zbpu_l2g  SetiL0=on  InitialCurrent=ini.iL_c  Capacitance=T.C*T.Zbpu_l2g  Setx0=on  InitialVoltage=ini.vC_c  Measurements=None
  A : PMIOPort  Side=Left
  B : PMIOPort  Port=2  Side=Left
  C : PMIOPort  Port=3  Side=Left
  connections:
  RLC1/LConn1 -- A/RConn1
  RLC2/LConn1 -- B/RConn1
  RLC3/LConn1 -- C/RConn1
  RLC1/RConn1 -- RLC3/RConn1 -- RLC2/RConn1

== system myLibrary/RL_line ==
  Series RLC Branch6 : spsSeriesRLCBranchLib/Series RLC Branch  LConnTagsString=__new0  RConnTagsString=__new0  BranchType=RL  Resistance=T.R  Inductance=T.L  SetiL0=on  InitialCurrent=ini.Ia  Capacitance=P.C  Setx0=on  InitialVoltage=P.C  Measurements=None
  Series RLC Branch7 : spsSeriesRLCBranchLib/Series RLC Branch  LConnTagsString=__new0  RConnTagsString=__new0  BranchType=RL  Resistance=T.R  Inductance=T.L  SetiL0=on  InitialCurrent=ini.Ic  Capacitance=P.C  Setx0=on  InitialVoltage=P.C  Measurements=None
  Series RLC Branch8 : spsSeriesRLCBranchLib/Series RLC Branch  LConnTagsString=__new0  RConnTagsString=__new0  BranchType=RL  Resistance=T.R  Inductance=T.L  SetiL0=on  InitialCurrent=ini.Ib  Capacitance=P.C  Setx0=on  InitialVoltage=P.C  Measurements=None
  A1 : PMIOPort  Side=Left
  B1 : PMIOPort  Port=2  Side=Left
  C1 : PMIOPort  Port=3  Side=Left
  A2 : PMIOPort  Port=4  Side=Right
  B2 : PMIOPort  Port=5  Side=Right
  C2 : PMIOPort  Port=6  Side=Right
  connections:
  C2/RConn1 -- Series RLC Branch7/RConn1
  Series RLC Branch7/LConn1 -- C1/RConn1
  B1/RConn1 -- Series RLC Branch8/LConn1
  B2/RConn1 -- Series RLC Branch8/RConn1
  A2/RConn1 -- Series RLC Branch6/RConn1
  A1/RConn1 -- Series RLC Branch6/LConn1

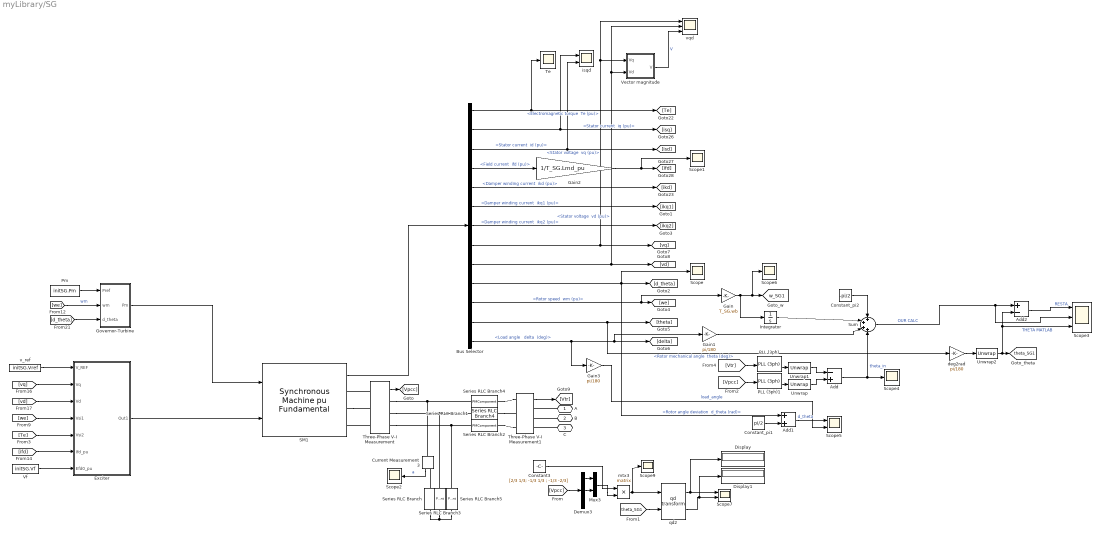
== system myLibrary/SG ==
  Add : Sum  Inputs=-+
  Add1 : Sum
  Add2 : Sum  Inputs=+-
  Bus Selector : BusSelector  OutputSignals="Mechanical.Electromagnetic torque  Te (pu),dq0 components.Stator current  iq (pu),dq0 components.Stator current  id (pu),dq0 components.Field current  ifd (pu),dq0 components.Damper winding current  ikd (pu),dq0 components.Damper winding current  ikq1 (pu),dq0 components.Damper winding current  ikq2 (pu),dq0 components.Stator voltage  vq (pu),dq0 components.Stator voltage  vd (pu),Mechanical.Rotor angle deviation  d_theta (rad),Mechanical.Rotor speed  wm (pu),Mechanical.Rotor mechanical angle  theta (deg),Load angle   delta  (deg)"
  Constant3 : Constant  Value=[2/3 1/3; -1/3 1/3 ; -1/3 -2/3]
  Constant_pi1 : Constant  Value=pi/2
  Constant_pi2 : Constant  Value=-pi/2
  Current Measurement3 : spsCurrentMeasurementLib/Current Measurement  PhasorSimulation=off  OutputType=Complex  PSBequivalent=0
  Demux3 : Demux  Outputs=3
  Display : Display
  Display1 : Display
  Exciter : Subsystem
  Gain : Gain  Gain=T_SG.wb
  Gain1 : Gain  Gain=pi/180
  Gain2 : Gain  Gain=1/T_SG.Lmd_pu
  Gain3 : Gain  Gain=pi/180
  Governor-Turbine : Subsystem
  Integrator : Integrator
  Mux3 : Mux  Inputs=2
  PLL (3ph) : spsPLL3phLib/PLL (3ph)  Fmin=45  Par_Init=[0, 50]  ParK=[180, 3200, 1]  TcD=1e-4  MaxRateChangeFreq=12  FilterCutOffFreq=25  Ts=0  AGC=on
  PLL (3ph)1 : spsPLL3phLib/PLL (3ph)  Fmin=45  Par_Init=[initSG.theta_in, 50]  ParK=[180, 3200, 1]  TcD=1e-4  MaxRateChangeFreq=12  FilterCutOffFreq=25  Ts=0  AGC=on
  Pm : Constant  Value=initSG.Pm
  SM1 : spsSynchronousMachinepuFundamentalLib/Synchronous Machine pu Fundamental  PresetModel=No  MechanicalLoad=Mechanical power Pm  ShowDetailedParameters=on  RotorType=Round  Units=per unit fundamental parameters  MeasurementBus=off  NominalParameters=initMachineBlocks{SGnum,1}  Stator=initMachineBlocks{SGnum,2}  Field=initMachineBlocks{SGnum,3}  Dampers2=initMachineBlocks{SGnum,4}  Dampers1="[ Rkd_pu   Llkd_pu  Rkq1_pu  Llkq1_pu]"  Mechanical=initMachineBlocks{SGnum,5}  PolePairs=1  InitialConditions=initMachineBlocks{SGnum,6}  SetSaturation=off  Saturation=[0.6404,0.7127,0.8441,0.9214,0.9956,1.082,1.19,1.316,1.457;0.7,0.7698,0.8872,0.9466,0.9969,1.046,1.1,1.151,1.201]  LoadFlowParameters=[1 5.55 0 0 0]  TsPowergui=0  TsBlock=-1  IterativeModel=Trapezoidal non iterative  IterativeDiscreteModel=Trapezoidal non iterative  BusType=PV  Pref=5.55  Qref=0  Qmin=-Inf  Qmax=Inf  PLF=0  QLF=0
  Scope{,1..2,4,6,9} (6 alike) : Scope
  Scope3 : Scope  NumInputPorts=3
  Scope5 : Scope  NumInputPorts=2
  Scope7 : Scope  NumInputPorts=2
  Series RLC Branch : spsSeriesRLCBranchLib/Series RLC Branch  LConnTagsString=__new0  RConnTagsString=__new0  BranchType=R  Resistance=T_SG.Rsnb*T_SG.Zbpu_l2g  Inductance=1e-3  SetiL0=off  InitialCurrent=0  Capacitance=1e-6  Setx0=off  InitialVoltage=0  Measurements=None
  Series RLC Branch1 : $bdroot/SG/Series RLC Branch4  LConnTagsString=__new0  RConnTagsString=__new0  BranchType=RL  Resistance=T_SG.Rtr*T_SG.Zbpu_l2g  Inductance=T_SG.Ltr*T_SG.Zbpu_l2g  SetiL0=off  InitialCurrent=initSG.Itr  Capacitance=P.C  Setx0=on  InitialVoltage=P.C  Measurements=None
      settings: LibrarySourceBlock=spsSeriesRLCBranchLib/Series RLC Branch
  Series RLC Branch2 : PMComponent  DialogController=POWERSYS.PowerSysDialog  LoadFcn=sps_rtmsupport('LoadFcn',gcbh);  StartFcn=sps_rtmsupport('StartFcn',gcbh);  StopFcn=sps_rtmsupport('StopFcn',gcbh);  PhysicalDomain=powersysdomain  LeftPortType=p1  RightPortType=p1  LConnTagsString=__new0  RConnTagsString=__new0  mask(Series RLC Branch){BranchType=RL, Resistance=T_SG.Rtr*T_SG.Zbpu_l2g, Inductance=T_SG.Ltr*T_SG.Zbpu_l2g, SetiL0=off, InitialCurrent=initSG.Itr, Capacitance=P.C, Setx0=on, InitialVoltage=P.C, Measurements=None}
      mask prompts: BranchType "Branch type:"; Resistance "Resistance (Ohms):"; Inductance "Inductance (H):"; SetiL0 "Set the initial inductor current"; InitialCurrent "Inductor initial current (A):"; Capacitance "Capacitance (F):"; Setx0 "Set the initial capacitor voltage"; InitialVoltage "Capacitor initial voltage (V):"
      mask help:
      | Implements a series branch of RLC elements.
      | Use the 'Branch type' parameter to add or remove elements from the branch.
      mask init:
      | [s1,s2,s3,s4,r1,r2,l1,l2,c1,c2,c3,c4] = powericon('Series RLC Branch',Resistance,Inductance,Capacitance,BranchType);
      | powericon('RLCCback',gcb)
      | power_initmask();
      settings: LibrarySourceBlock=spsSeriesRLCBranchLib/Series RLC Branch  CopyFcn=sps_rtmsupport('CopyFcn',gcbh);  DeleteFcn=sps_rtmsupport('DeleteFcn',gcbh);  UndoDeleteFcn=sps_rtmsupport('UndoDeleteFcn',gcbh);  ModelCloseFcn=sps_rtmsupport('ModelCloseFcn',gcbh);  PreSaveFcn=sps_rtmsupport('PreSaveFcn',gcbh);  PostSaveFcn=sps_rtmsupport('PostSaveFcn',gcbh);  NameChangeFcn=sps_rtmsupport('NameChangeFcn',gcbh);  PreCopyFcn=sps_rtmsupport('PreCopyFcn',gcbh);  OpenFcn=sps_rtmsupport('OpenFcn',gcbh, [1 4 7 9]);  CloseFcn=sps_rtmsupport('CloseFcn',gcbh);  PreDeleteFcn=sps_rtmsupport('PreDeleteFcn',gcbh);
      mask Help: helpview(psbhelp);
      mask TypeOptions BranchType: RLC | R | L | C | RL | RC | LC | Open circuit
      mask Callback BranchType: powericon('RLCCback',gcb)
      mask Callback Resistance: powericon('RLCCback',gcb)
      mask Callback Inductance: powericon('RLCCback',gcb)
      mask Callback SetiL0: powericon('RLCCback',gcb)
      mask Callback Capacitance: powericon('RLCCback',gcb)
      mask Callback Setx0: powericon('RLCCback',gcb)
      mask TypeOptions Measurements: None | Branch voltage | Branch current | Branch voltage and current
      mask Display:
      | plot(s1,s2,s3,s4,r1,r2*1.5,l1,l2*1.5,c1,c2*1.5,c3,c4*1.5)
      | color('red')
      | port_label('LConn',1,'+')
  Series RLC Branch3 : PMComponent  DialogController=POWERSYS.PowerSysDialog  LoadFcn=sps_rtmsupport('LoadFcn',gcbh);  StartFcn=sps_rtmsupport('StartFcn',gcbh);  StopFcn=sps_rtmsupport('StopFcn',gcbh);  PhysicalDomain=powersysdomain  LeftPortType=p1  RightPortType=p1  LConnTagsString=__new0  RConnTagsString=__new0  mask(Series RLC Branch){BranchType=R, Resistance=T_SG.Rsnb*T_SG.Zbpu_l2g, Inductance=1e-3, SetiL0=off, InitialCurrent=0, Capacitance=1e-6, Setx0=off, InitialVoltage=0, Measurements=None}
      mask prompts: BranchType "Branch type:"; Resistance "Resistance (Ohms):"; Inductance "Inductance (H):"; SetiL0 "Set the initial inductor current"; InitialCurrent "Inductor initial current (A):"; Capacitance "Capacitance (F):"; Setx0 "Set the initial capacitor voltage"; InitialVoltage "Capacitor initial voltage (V):"
      mask help:
      | Implements a series branch of RLC elements.
      | Use the 'Branch type' parameter to add or remove elements from the branch.
      mask init:
      | [s1,s2,s3,s4,r1,r2,l1,l2,c1,c2,c3,c4] = powericon('Series RLC Branch',Resistance,Inductance,Capacitance,BranchType);
      | powericon('RLCCback',gcb)
      | power_initmask();
      settings: LibrarySourceBlock=sps_lib/Passives/Series RLC Branch  CopyFcn=sps_rtmsupport('CopyFcn',gcbh);  DeleteFcn=sps_rtmsupport('DeleteFcn',gcbh);  UndoDeleteFcn=sps_rtmsupport('UndoDeleteFcn',gcbh);  ModelCloseFcn=sps_rtmsupport('ModelCloseFcn',gcbh);  PreSaveFcn=sps_rtmsupport('PreSaveFcn',gcbh);  PostSaveFcn=sps_rtmsupport('PostSaveFcn',gcbh);  NameChangeFcn=sps_rtmsupport('NameChangeFcn',gcbh);  PreCopyFcn=sps_rtmsupport('PreCopyFcn',gcbh);  OpenFcn=sps_rtmsupport('OpenFcn',gcbh, [1 4 7 9]);  CloseFcn=sps_rtmsupport('CloseFcn',gcbh);  PreDeleteFcn=sps_rtmsupport('PreDeleteFcn',gcbh);
      mask Help: helpview(psbhelp);
      mask TypeOptions BranchType: RLC | R | L | C | RL | RC | LC | Open circuit
      mask Callback BranchType: powericon('RLCCback',gcb)
      mask Callback Resistance: powericon('RLCCback',gcb)
      mask Callback Inductance: powericon('RLCCback',gcb)
      mask Callback SetiL0: powericon('RLCCback',gcb)
      mask Callback Capacitance: powericon('RLCCback',gcb)
      mask Callback Setx0: powericon('RLCCback',gcb)
      mask TypeOptions Measurements: None | Branch voltage | Branch current | Branch voltage and current
      mask Display:
      | plot(s1,s2,s3,s4,r1,r2*1.5,l1,l2*1.5,c1,c2*1.5,c3,c4*1.5)
      | color('red')
      | port_label('LConn',1,'+')
  Series RLC Branch4 : PMComponent  DialogController=POWERSYS.PowerSysDialog  LoadFcn=sps_rtmsupport('LoadFcn',gcbh);  StartFcn=sps_rtmsupport('StartFcn',gcbh);  StopFcn=sps_rtmsupport('StopFcn',gcbh);  PhysicalDomain=powersysdomain  LeftPortType=p1  RightPortType=p1  LConnTagsString=__new0  RConnTagsString=__new0  mask(Series RLC Branch){BranchType=RL, Resistance=T_SG.Rtr*T_SG.Zbpu_l2g, Inductance=T_SG.Ltr*T_SG.Zbpu_l2g, SetiL0=off, InitialCurrent=initSG.Itr, Capacitance=P.C, Setx0=on, InitialVoltage=P.C, Measurements=None}
      mask prompts: BranchType "Branch type:"; Resistance "Resistance (Ohms):"; Inductance "Inductance (H):"; SetiL0 "Set the initial inductor current"; InitialCurrent "Inductor initial current (A):"; Capacitance "Capacitance (F):"; Setx0 "Set the initial capacitor voltage"; InitialVoltage "Capacitor initial voltage (V):"
      mask help:
      | Implements a series branch of RLC elements.
      | Use the 'Branch type' parameter to add or remove elements from the branch.
      mask init:
      | [s1,s2,s3,s4,r1,r2,l1,l2,c1,c2,c3,c4] = powericon('Series RLC Branch',Resistance,Inductance,Capacitance,BranchType);
      | powericon('RLCCback',gcb)
      | power_initmask();
      settings: LibrarySourceBlock=spsSeriesRLCBranchLib/Series RLC Branch  CopyFcn=sps_rtmsupport('CopyFcn',gcbh);  DeleteFcn=sps_rtmsupport('DeleteFcn',gcbh);  UndoDeleteFcn=sps_rtmsupport('UndoDeleteFcn',gcbh);  ModelCloseFcn=sps_rtmsupport('ModelCloseFcn',gcbh);  PreSaveFcn=sps_rtmsupport('PreSaveFcn',gcbh);  PostSaveFcn=sps_rtmsupport('PostSaveFcn',gcbh);  NameChangeFcn=sps_rtmsupport('NameChangeFcn',gcbh);  PreCopyFcn=sps_rtmsupport('PreCopyFcn',gcbh);  OpenFcn=sps_rtmsupport('OpenFcn',gcbh, [1 4 7 9]);  CloseFcn=sps_rtmsupport('CloseFcn',gcbh);  PreDeleteFcn=sps_rtmsupport('PreDeleteFcn',gcbh);
      mask Help: helpview(psbhelp);
      mask TypeOptions BranchType: RLC | R | L | C | RL | RC | LC | Open circuit
      mask Callback BranchType: powericon('RLCCback',gcb)
      mask Callback Resistance: powericon('RLCCback',gcb)
      mask Callback Inductance: powericon('RLCCback',gcb)
      mask Callback SetiL0: powericon('RLCCback',gcb)
      mask Callback Capacitance: powericon('RLCCback',gcb)
      mask Callback Setx0: powericon('RLCCback',gcb)
      mask TypeOptions Measurements: None | Branch voltage | Branch current | Branch voltage and current
      mask Display:
      | plot(s1,s2,s3,s4,r1,r2*1.5,l1,l2*1.5,c1,c2*1.5,c3,c4*1.5)
      | color('red')
      | port_label('LConn',1,'+')
  Series RLC Branch5 : PMComponent  DialogController=POWERSYS.PowerSysDialog  LoadFcn=sps_rtmsupport('LoadFcn',gcbh);  StartFcn=sps_rtmsupport('StartFcn',gcbh);  StopFcn=sps_rtmsupport('StopFcn',gcbh);  PhysicalDomain=powersysdomain  LeftPortType=p1  RightPortType=p1  LConnTagsString=__new0  RConnTagsString=__new0  mask(Series RLC Branch){BranchType=R, Resistance=T_SG.Rsnb*T_SG.Zbpu_l2g, Inductance=1e-3, SetiL0=off, InitialCurrent=0, Capacitance=1e-6, Setx0=off, InitialVoltage=0, Measurements=None}
      mask prompts: BranchType "Branch type:"; Resistance "Resistance (Ohms):"; Inductance "Inductance (H):"; SetiL0 "Set the initial inductor current"; InitialCurrent "Inductor initial current (A):"; Capacitance "Capacitance (F):"; Setx0 "Set the initial capacitor voltage"; InitialVoltage "Capacitor initial voltage (V):"
      mask help:
      | Implements a series branch of RLC elements.
      | Use the 'Branch type' parameter to add or remove elements from the branch.
      mask init:
      | [s1,s2,s3,s4,r1,r2,l1,l2,c1,c2,c3,c4] = powericon('Series RLC Branch',Resistance,Inductance,Capacitance,BranchType);
      | powericon('RLCCback',gcb)
      | power_initmask();
      settings: LibrarySourceBlock=sps_lib/Passives/Series RLC Branch  CopyFcn=sps_rtmsupport('CopyFcn',gcbh);  DeleteFcn=sps_rtmsupport('DeleteFcn',gcbh);  UndoDeleteFcn=sps_rtmsupport('UndoDeleteFcn',gcbh);  ModelCloseFcn=sps_rtmsupport('ModelCloseFcn',gcbh);  PreSaveFcn=sps_rtmsupport('PreSaveFcn',gcbh);  PostSaveFcn=sps_rtmsupport('PostSaveFcn',gcbh);  NameChangeFcn=sps_rtmsupport('NameChangeFcn',gcbh);  PreCopyFcn=sps_rtmsupport('PreCopyFcn',gcbh);  OpenFcn=sps_rtmsupport('OpenFcn',gcbh, [1 4 7 9]);  CloseFcn=sps_rtmsupport('CloseFcn',gcbh);  PreDeleteFcn=sps_rtmsupport('PreDeleteFcn',gcbh);
      mask Help: helpview(psbhelp);
      mask TypeOptions BranchType: RLC | R | L | C | RL | RC | LC | Open circuit
      mask Callback BranchType: powericon('RLCCback',gcb)
      mask Callback Resistance: powericon('RLCCback',gcb)
      mask Callback Inductance: powericon('RLCCback',gcb)
      mask Callback SetiL0: powericon('RLCCback',gcb)
      mask Callback Capacitance: powericon('RLCCback',gcb)
      mask Callback Setx0: powericon('RLCCback',gcb)
      mask TypeOptions Measurements: None | Branch voltage | Branch current | Branch voltage and current
      mask Display:
      | plot(s1,s2,s3,s4,r1,r2*1.5,l1,l2*1.5,c1,c2*1.5,c3,c4*1.5)
      | color('red')
      | port_label('LConn',1,'+')
  Sum : Sum  Inputs=++++
  Te : Scope
  Three-Phase V-I Measurement : spsThreePhaseVIMeasurementLib/Three-Phase V-I Measurement  VoltageMeasurement=phase-to-phase  SetLabelV=off  LabelV=Vpcc  Vpu=off  VpuLL=off  CurrentMeasurement=no  SetLabelI=off  LabelI=Iabc  Ipu=off  Pbase=100e6  Vbase=500e3  OutputType=Complex  PhasorSimulation=off  PSBequivalent=0
  Three-Phase V-I Measurement1 : spsThreePhaseVIMeasurementLib/Three-Phase V-I Measurement  VoltageMeasurement=phase-to-phase  SetLabelV=off  LabelV=Vtr  Vpu=off  VpuLL=off  CurrentMeasurement=no  SetLabelI=off  LabelI=Iabc  Ipu=off  Pbase=100e6  Vbase=500e3  OutputType=Complex  PhasorSimulation=off  PSBequivalent=0
  Unwrap : dspsigops/Unwrap  tol=pi  InputProcessing=Columns as channels (frame based)  running=off
  Unwrap1 : dspsigops/Unwrap  tol=pi  InputProcessing=Columns as channels (frame based)  running=off
  Unwrap2 : dspsigops/Unwrap  tol=pi  InputProcessing=Columns as channels (frame based)  running=off
  "Vector magnitude " : Subsystem
  Vf : Constant  Value=initSG.Vf
  deg2rad : Gain  Gain=pi/180
  isqd : Scope  NumInputPorts=2
  mtx3 : Product  Multiplication=Matrix(*)
  qd2 : $bdroot/qd transform  SystemSampleTime=-1  VariantActivationTime=update diagram  AllowFlexibleInterface=on  Latency=0  AutoFrameSizeCalculation=off
  v_ref : Constant  Value=initSG.Vref
  vqd : Scope  NumInputPorts=3
  A : PMIOPort  Side=Right
  B : PMIOPort  Port=2  Side=Right
  C : PMIOPort  Port=3  Side=Right
  tag scope: theta_SG1=global, w_SG1=global
  wires:
  Three-Phase V-I Measurement1/1 -> [Vtr]
  Three-Phase V-I Measurement/1 -> [Vpcc]
  Bus Selector/10 -> [d_theta], Add1/1, Scope/1  "<Rotor angle deviation  d_theta (rad)>"
  Bus Selector/7 -> [ikq2]  "<Damper winding current  ikq2 (pu)>"
  [Vtr] -> PLL (3ph)/1
  Gain2/1 -> Scope1/1, [ifd]
  Bus Selector/5 -> [ikd]  "<Damper winding current  ikd (pu)>"
  Bus Selector/3 -> isqd/2, [isd]  "<Stator current  id (pu)>"
  Bus Selector/11 -> [we], Gain/1  "<Rotor speed  wm (pu)>"
  Bus Selector/6 -> [ikq1]  "<Damper winding current  ikq1 (pu)>"
  [Vpcc] -> PLL (3ph)1/1
  Bus Selector/4 -> Gain2/1  "<Field current  ifd (pu)>"
  Bus Selector/8 -> "Vector magnitude "/1(Vq), vqd/1, [vq]  "<Stator voltage  vq (pu)>"
  Bus Selector/1 -> Te/1, [Te]  "<Electromagnetic torque  Te (pu)>"
  Bus Selector/9 -> "Vector magnitude "/2(Vd), vqd/2, [vd]  "<Stator voltage  vd (pu)>"
  Gain/1 -> Scope6/1, [w_SG1], Integrator/1
  Current Measurement3/1 -> Scope2/1  "a"
  "Vector magnitude "/1(V) -> vqd/3  "V"
  Unwrap1/1 -> Add/1
  SM1/1 -> Bus Selector/1
  Bus Selector/13 -> [delta], Gain1/1, Gain3/1  "<Load angle   delta  (deg)>"
  Bus Selector/12 -> deg2rad/1, [theta]  "<Rotor mechanical angle  theta (deg)>"
  Bus Selector/2 -> isqd/1, [isq]  "<Stator current  iq (pu)>"
  Add/1 -> Scope4/1, Sum/4  "theta_in"
  Integrator/1 -> Sum/2
  PLL (3ph)1/2 -> Unwrap/1
  PLL (3ph)/2 -> Unwrap1/1
  Unwrap/1 -> Add/2
  Constant_pi1/1 -> Add1/2
  Add1/1 -> Scope5/1  "d_theta"
  Gain3/1 -> Scope5/2  "load_angle"
  Gain1/1 -> Sum/3
  Constant_pi2/1 -> Sum/1
  Governor-Turbine/1(Pm) -> SM1/1
  [we] -> Governor-Turbine/2(wm)  "wm"
  Pm/1 -> Governor-Turbine/1(Pref)
  [d_theta] -> Governor-Turbine/3(d_theta)
  deg2rad/1 -> Unwrap2/1
  Unwrap2/1 -> Add2/2, Scope3/3, [theta_SG1]  "THETA MATLAB"
  [we] -> Exciter/4(Vsi1)
  [vd] -> Exciter/3(Vd)
  [ifd] -> Exciter/6(Ifd_pu)
  [Te] -> Exciter/5(Vsi2)
  Vf/1 -> Exciter/7(Efd0_pu)
  v_ref/1 -> Exciter/1(V_REF)
  Exciter/1(Out1) -> SM1/2
  [vq] -> Exciter/2(Vq)
  Sum/1 -> Scope3/2, Add2/1  "OUR CALC"
  Add2/1 -> Scope3/1  "RESTA"
  Demux3/2 -> Mux3/2
  [Vpcc] -> Demux3/1
  Demux3/1 -> Mux3/1
  Mux3/1 -> mtx3/2
  Constant3/1 -> mtx3/1
  mtx3/1 -> qd2/1, Scope9/1
  [theta_SG1] -> qd2/2
  qd2/1 -> Display/1, Scope7/1
  qd2/2 -> Display1/1, Scope7/2
  connections:
  Three-Phase V-I Measurement/LConn3 -- SM1/RConn3
  SM1/RConn2 -- Three-Phase V-I Measurement/LConn2
  Three-Phase V-I Measurement/LConn1 -- SM1/RConn1
  B/RConn1 -- Three-Phase V-I Measurement1/RConn2
  Series RLC Branch2/RConn1 -- Three-Phase V-I Measurement1/LConn3
  Series RLC Branch4/RConn1 -- Three-Phase V-I Measurement1/LConn1
  Series RLC Branch/LConn1 -- Current Measurement3/RConn1
  A/RConn1 -- Three-Phase V-I Measurement1/RConn1
  C/RConn1 -- Three-Phase V-I Measurement1/RConn3
  Series RLC Branch1/RConn1 -- Three-Phase V-I Measurement1/LConn2
  Three-Phase V-I Measurement/RConn1 -- Series RLC Branch4/LConn1 -- Current Measurement3/LConn1
  Three-Phase V-I Measurement/RConn3 -- Series RLC Branch2/LConn1 -- Series RLC Branch5/LConn1
  Series RLC Branch/RConn1 -- Series RLC Branch5/RConn1 -- Series RLC Branch3/RConn1
  Three-Phase V-I Measurement/RConn2 -- Series RLC Branch1/LConn1 -- Series RLC Branch3/LConn1
